simulink library "waveFlow_ul"  (R2018b)
settings: Solver=VariableStepAuto  StartTime=0.0  StopTime=10.0  RelTol=1e-3
undefined symbols (not defined in the file or in its folder): e
settings Model: Creator=mcobb  LastModifiedBy=MAE-NCSUCORE

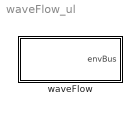
== system waveFlow_ul ==
  waveFlow : Subsystem  mask{e=e}
      mask prompts: e "Environment Object"

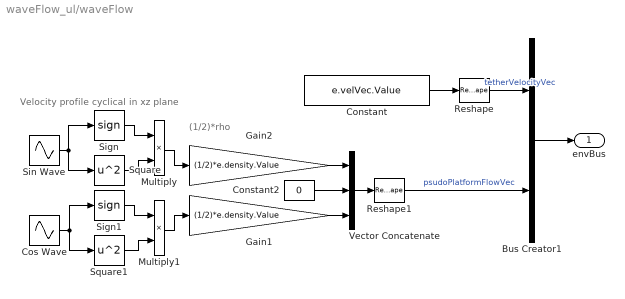
== system waveFlow_ul/waveFlow ==
  note: (1/2)*rho
  note: Velocity profile cyclical
      | in xz plane
  Bus Creator1 : BusCreator  Inputs=2  OutDataTypeStr=Bus:envBus
  Constant : Constant  Value=e.velVec.Value
  Constant2 : Constant  Value=0
  Cos Wave : Sin  Amplitude=e.pltfrmAppFlwMag.Value  Frequency=2*pi*e.wavePeriod  Phase=pi/2  SampleTime=0
  Gain1 : Gain  Gain=(1/2)*e.density.Value
  Gain2 : Gain  Gain=(1/2)*e.density.Value
  Multiply : Product
  Multiply1 : Product
  Reshape : Reshape  OutputDimensionality=Column vector (2-D)
  Reshape1 : Reshape  OutputDimensionality=Column vector (2-D)
  Sign : Signum
  Sign1 : Signum
  Sin Wave : Sin  Amplitude=e.pltfrmAppFlwMag.Value  Frequency=2*pi*e.wavePeriod  SampleTime=0
  Square : Math  Operator=square  SaturateOnIntegerOverflow=on
  Square1 : Math  Operator=square  SaturateOnIntegerOverflow=on
  Vector Concatenate : Concatenate  NumInputs=3
  envBus : Outport  OutDataTypeStr=Bus: envBus
  wires:
  Bus Creator1/1 -> envBus/1
  Constant/1 -> Reshape/1
  Reshape/1 -> Bus Creator1/1  "tetherVelocityVec"
  Reshape1/1 -> Bus Creator1/2  "psudoPlatformFlowVec"
  Vector Concatenate/1 -> Reshape1/1
  Constant2/1 -> Vector Concatenate/2
  Gain1/1 -> Vector Concatenate/3
  Gain2/1 -> Vector Concatenate/1
  Sin Wave/1 -> Square/1, Sign/1
  Multiply/1 -> Gain2/1
  Square/1 -> Multiply/2
  Sign/1 -> Multiply/1
  Sign1/1 -> Multiply1/1
  Square1/1 -> Multiply1/2
  Multiply1/1 -> Gain1/1
  Cos Wave/1 -> Sign1/1, Square1/1
